simulink model "simcape_real_time_V2"  (R2022b)
settings: Solver=ode8  StartTime=0.0  StopTime=100  FixedStep=0.002  RelTol=1e-3
undefined symbols (not defined in the file): drone_leg, K_LQR, K_LQR_GOC, pitch_init, roll_init, v_pitch_init, v_roll_init, v_x_init, v_y_init, v_yaw_init, v_z_init, X, x_init, Y, y_init, yaw_init, Z, z_init
libraries: sm_lib x55, nesl_utility x12, simulink x7
(part 3 of 3)

== system simcape_real_time_V2/Subsystem4 ==
  Constant : Constant  Value=10
  Display : Display
  Subsystem : Subsystem
  Subsystem1 : Subsystem
  Subsystem3 : Subsystem
  Roll SP : Outport
  Pitch SP : Outport  Port=2
  wires:
  Subsystem/1(U1) -> Subsystem1/1(U1)
  Subsystem3/2(Pitch SP) -> Pitch SP/1
  Subsystem3/1(Roll SP) -> Roll SP/1
  [X_y] -> Subsystem1/3(y_SP)
  [X_x] -> Subsystem1/2(x_SP)
  Constant/1 -> Subsystem/1(z_SP)

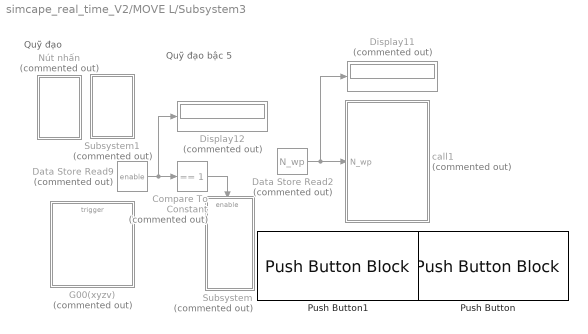
== system simcape_real_time_V2/MOVE L/Subsystem3 ==
  note: Quỹ đạo bậc 5
  note: Quỹ đạo
  Compare To Constant : simulink/Logic and Bit Operations/Compare To Constant  Commented=on  relop===  const=1  OutDataTypeStr=boolean
  Data Store Read2 : DataStoreRead  Commented=on  DataStoreName=N_wp  DataStoreElements=N_wp  IndexOptions=Index vector (dialog)  Indices=1  OutputSizes=1
  Data Store Read9 : DataStoreRead  Commented=on  DataStoreName=enable  IndexOptions=Index vector (dialog)  Indices=1  OutputSizes=1
  Display11 : Display  Commented=on
  Display12 : Display  Commented=on
  G00(xyzv) : Subsystem  Commented=on  TreatAsAtomicUnit=on
  Nút nhấn : Subsystem  Commented=on
  Push Button : PushButtonBlock  ButtonText=Start  IconColor=On  OffValue=0.000000
  Push Button1 : PushButtonBlock  ButtonText=Stop  IconColor=On  OffValue=0.000000
  Subsystem : Subsystem  Commented=on
  Subsystem1 : Subsystem  Commented=on
  call1 : MATLAB Function  Commented=on  TreatAsAtomicUnit=on
  wires:
  Data Store Read9/1 -> Display12/1, Compare To Constant/1
  Data Store Read2/1 -> Display11/1, call1/1(N_wp)
  Compare To Constant/1 -> Subsystem/Enable

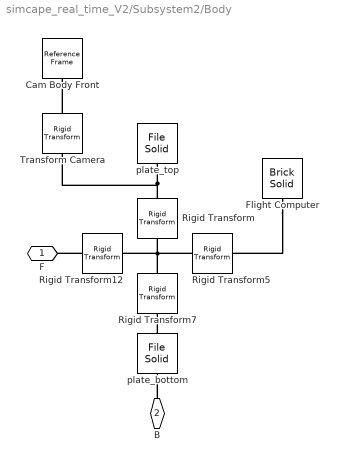
== system simcape_real_time_V2/Subsystem2/Body ==
  Cam Body Front : sm_lib/Frames and Transforms/Reference Frame
  Flight Computer : sm_lib/Body Elements/Brick Solid  GraphicAmbientColor=[0.15 0.15 0.15 1.0]  BasedOnType=Mass  BrickDimensions=3*[20 20 5]  BrickDimensionUnits=mm  CenterOfMass=[0 0 0]  CenterOfMassUnits=m  GraphicDiffuseColor=[0.5 0.5 0.5]  Density=1000  DensityUnits=kg/m^3  DoExposeReferenceFrame=on  GraphicEmissiveColor=[0.0 0.0 0.0 1.0]  ExportEntireGeometry=off  SerializedFrames=<Frames/>  MarkerShape=Sphere  MarkerSize=10  GraphicType=FromGeometry  InertiaType=CalculateFromGeometry  Mass=638  MassUnits=g  MomentsOfInertia=[1 1 1]  MomentsOfInertiaUnits=kg*m^2  GraphicOpacity=1.0  ProductsOfInertia=[0 0 0]  ProductsOfInertiaUnits=kg*m^2  GraphicShininess=75  GraphicSpecularColor=[0.5 0.5 0.5 1.0]  GraphicVisPropType=SimpleVisualProperties
  Rigid Transform : sm_lib/Frames and Transforms/Rigid Transform  TranslationMethod=None  TranslationStandardOffset=0  TranslationLengthUnit=m  TranslationStandardAxis=+Z  TranslationCartesianOffset=[0 0 0]  TranslationROffset=0  TranslationROffsetUnits=m  TranslationZOffset=0  TranslationZOffsetUnits=m  TranslationThetaOffset=0  TranslationThetaOffsetUnits=deg  RotationMethod=None  RotationAngleUnits=deg  RotationStandardAxis=+Z  RotationAngle=45  RotationArbitraryAxis=[0 0 1]  FollAlignAxisA=+X  BaseAlignAxisA=+Y  FollAlignAxisB=+Y  BaseAlignAxisB=+Z  RotationSequenceAxes=FollowerAxes  RotationSequence=XYX  RotationSequenceAngles=[0 0 0]  RotationSequenceAnglesUnits=deg  RotationMatrix=[1 0 0; 0 1 0; 0 0 1]  Quaternion=[1 0 0 0]
  Rigid Transform12 : sm_lib/Frames and Transforms/Rigid Transform  TranslationMethod=Cartesian  TranslationStandardOffset=0  TranslationLengthUnit=mm  TranslationStandardAxis=+Z  TranslationCartesianOffset=[0 0 -26]  TranslationROffset=0  TranslationROffsetUnits=m  TranslationZOffset=0  TranslationZOffsetUnits=m  TranslationThetaOffset=0  TranslationThetaOffsetUnits=deg  RotationMethod=None  RotationAngleUnits=deg  RotationStandardAxis=+Z  RotationAngle=45  RotationArbitraryAxis=[0 0 1]  FollAlignAxisA=+X  BaseAlignAxisA=+Y  FollAlignAxisB=+Y  BaseAlignAxisB=+Z  RotationSequenceAxes=FollowerAxes  RotationSequence=XYX  RotationSequenceAngles=[0 0 0]  RotationSequenceAnglesUnits=deg  RotationMatrix=[1 0 0; 0 1 0; 0 0 1]  Quaternion=[1 0 0 0]
  Rigid Transform5 : sm_lib/Frames and Transforms/Rigid Transform  TranslationMethod=Cartesian  TranslationStandardOffset=0  TranslationLengthUnit=mm  TranslationStandardAxis=+Z  TranslationCartesianOffset=[0 0 -26]  TranslationROffset=0  TranslationROffsetUnits=m  TranslationZOffset=0  TranslationZOffsetUnits=m  TranslationThetaOffset=0  TranslationThetaOffsetUnits=deg  RotationMethod=None  RotationAngleUnits=deg  RotationStandardAxis=+Z  RotationAngle=45  RotationArbitraryAxis=[0 0 1]  FollAlignAxisA=+X  BaseAlignAxisA=+Y  FollAlignAxisB=+Y  BaseAlignAxisB=+Z  RotationSequenceAxes=FollowerAxes  RotationSequence=XYX  RotationSequenceAngles=[0 0 0]  RotationSequenceAnglesUnits=deg  RotationMatrix=[1 0 0; 0 1 0; 0 0 1]  Quaternion=[1 0 0 0]
  Rigid Transform7 : sm_lib/Frames and Transforms/Rigid Transform  TranslationMethod=Cartesian  TranslationStandardOffset=0  TranslationLengthUnit=mm  TranslationStandardAxis=+Z  TranslationCartesianOffset=[0 0 -38]  TranslationROffset=0  TranslationROffsetUnits=m  TranslationZOffset=0  TranslationZOffsetUnits=m  TranslationThetaOffset=0  TranslationThetaOffsetUnits=deg  RotationMethod=None  RotationAngleUnits=deg  RotationStandardAxis=+Z  RotationAngle=45  RotationArbitraryAxis=[0 0 1]  FollAlignAxisA=+X  BaseAlignAxisA=+Y  FollAlignAxisB=+Y  BaseAlignAxisB=+Z  RotationSequenceAxes=FollowerAxes  RotationSequence=XYX  RotationSequenceAngles=[0 0 0]  RotationSequenceAnglesUnits=deg  RotationMatrix=[1 0 0; 0 1 0; 0 0 1]  Quaternion=[1 0 0 0]
  Transform Camera : sm_lib/Frames and Transforms/Rigid Transform  TranslationMethod=Cartesian  TranslationStandardOffset=0  TranslationLengthUnit=m  TranslationStandardAxis=+Z  TranslationCartesianOffset=[0.06 0 0]  TranslationROffset=0  TranslationROffsetUnits=m  TranslationZOffset=0  TranslationZOffsetUnits=m  TranslationThetaOffset=0  TranslationThetaOffsetUnits=deg  RotationMethod=None  RotationAngleUnits=deg  RotationStandardAxis=+Z  RotationAngle=0.0  RotationArbitraryAxis=[0 0 1]  FollAlignAxisA=+X  BaseAlignAxisA=+Y  FollAlignAxisB=+Y  BaseAlignAxisB=+Z  RotationSequenceAxes=FollowerAxes  RotationSequence=XYX  RotationSequenceAngles=[0 0 0]  RotationSequenceAnglesUnits=deg  RotationMatrix=[1 0 0; 0 1 0; 0 0 1]  Quaternion=[1 0 0 0]
  plate_bottom : sm_lib/Body Elements/File Solid  ExtGeomFileName=C:\Users\tridu\OneDrive\Máy tính\(1)\mohinh\quadcopter_simscape\Quadcopter-Simulation-master\Quadcopter-Simulation-master\CAD\Geometry\quadcopter_drone_plate_bottom.stp  UnitType=FromFile  ExtGeomFileUnits=m  StepReaderType=HEX  ExportConvexHullGeometry=off  InertiaType=Custom  Mass=0.0317292  MassUnits=kg  CenterOfMass=[9.57262e-08, 1.0716e-07, -1.47882e-10]  CenterOfMassUnits=m  MomentsOfInertia=[2.77785e-05, 2.75764e-05, 5.53432e-05]  MomentsOfInertiaUnits=kg*m^2  ProductsOfInertia=[-9.24719e-13, -9.71809e-13, 1.0181e-10]  ProductsOfInertiaUnits=kg*m^2  BasedOnType=Density  Density=1  DensityUnits=g/cm^3  DoExposeReferenceFrame=off  SerializedFrames=<Frames><Frame><Id>Frame1</Id><Value><Name>Bot</Name><Origin><Source>GeometricFeature</Source><FeatureName>planar surface 33</FeatureName></Origin><PrimaryAxis><DefinedDirection>+Z</DefinedDirection><Source>ReferenceFrame</Source><SourceDirection>+Z</SourceDirection><FeatureName></FeatureName></PrimaryAxis><SecondaryAxis><DefinedDirection>+X</DefinedDirection><Source>ReferenceFrame</Source><SourceDirection>+Y</SourceDirection><FeatureName></FeatureName></SecondaryAxis></Value></Frame><Frame><Id>Frame2</Id><Value><Name>Top</Name><Origin><Source>ReferenceFrame</Source><FeatureName></FeatureName></Origin><PrimaryAxis><DefinedDirection>+Z</DefinedDirection><Source>ReferenceFrame</Source><SourceDirection>+Z</SourceDirection><FeatureName></FeatureName></PrimaryAxis><SecondaryAxis><DefinedDirection>+X</DefinedDirection><Source>ReferenceFrame</Source><SourceDirection>+Y</SourceDirection><FeatureName></FeatureName></SecondaryAxis></Value></Frame></Frames>  GraphicType=FromGeometry  MarkerShape=Sphere  MarkerSize=10  GraphicVisPropType=SimpleVisualProperties  GraphicDiffuseColor=[0.0 0.0 0.0]  GraphicSpecularColor=[0.5 0.5 0.5 1.0]  GraphicAmbientColor=[0.15 0.15 0.15 1.0]  GraphicEmissiveColor=[0.0 0.0 0.0 1.0]  GraphicShininess=75  GraphicOpacity=1.0
  "plate_top " : sm_lib/Body Elements/File Solid  ExtGeomFileName=C:\Users\tridu\OneDrive\Máy tính\(1)\mohinh\quadcopter_simscape\Quadcopter-Simulation-master\Quadcopter-Simulation-master\CAD\Geometry\quadcopter_drone_plate_top.stp  UnitType=FromFile  ExtGeomFileUnits=m  StepReaderType=HEX  ExportConvexHullGeometry=off  InertiaType=Custom  Mass=0.0317292  MassUnits=kg  CenterOfMass=[9.57262e-08, 1.0716e-07, -1.47882e-10]  CenterOfMassUnits=m  MomentsOfInertia=[2.77785e-05, 2.75764e-05, 5.53432e-05]  MomentsOfInertiaUnits=kg*m^2  ProductsOfInertia=[-9.24719e-13, -9.71809e-13, 1.0181e-10]  ProductsOfInertiaUnits=kg*m^2  BasedOnType=Density  Density=1  DensityUnits=g/cm^3  DoExposeReferenceFrame=on  SerializedFrames=<Frames/>  GraphicType=FromGeometry  MarkerShape=Sphere  MarkerSize=10  GraphicVisPropType=SimpleVisualProperties  GraphicDiffuseColor=[0.0 0.0 0.0]  GraphicSpecularColor=[0.5 0.5 0.5 1.0]  GraphicAmbientColor=[0.15 0.15 0.15 1.0]  GraphicEmissiveColor=[0.0 0.0 0.0 1.0]  GraphicShininess=75  GraphicOpacity=1.0
  F : PMIOPort  Side=Right
  B : PMIOPort  Port=2  Side=Left
  connections:
  Flight Computer/RConn1 -- Rigid Transform5/RConn1
  Rigid Transform7/LConn1 -- Rigid Transform5/LConn1 -- Rigid Transform12/LConn1 -- Rigid Transform/LConn1
  plate_bottom/RConn1 -- Rigid Transform7/RConn1
  Rigid Transform12/RConn1 -- F/RConn1
  Rigid Transform/RConn1 -- Transform Camera/LConn1 -- "plate_top "/RConn1
  Transform Camera/RConn1 -- Cam Body Front/RConn1
  B/RConn1 -- plate_bottom/LConn1

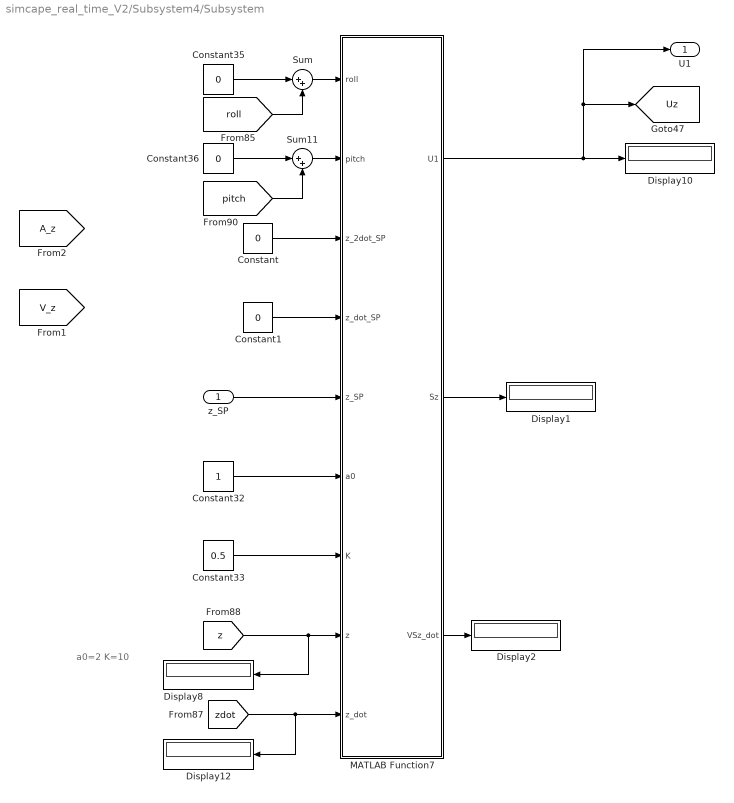
== system simcape_real_time_V2/Subsystem4/Subsystem ==
  note: a0=2
      | K=10
  z_SP : Inport
  Constant{,1,35..36} (4 alike) : Constant  Value=0
  Constant32 : Constant
  Constant33 : Constant  Value=0.5
  Display{1..2,8,10,12} (5 alike) : Display
  MATLAB Function7 : MATLAB Function  TreatAsAtomicUnit=on
  Sum : Sum  Inputs=|++
  Sum11 : Sum  Inputs=|++
  U1 : Outport
  tag scope: Uz=global
  wires:
  [z] -> Display8/1, MATLAB Function7/8(z)
  Constant35/1 -> Sum/1
  Constant32/1 -> MATLAB Function7/6(a0)
  [zdot] -> Display12/1, MATLAB Function7/9(z_dot)
  Sum11/1 -> MATLAB Function7/2(pitch)
  [roll] -> Sum/2
  Constant33/1 -> MATLAB Function7/7(K)
  [pitch] -> Sum11/2
  Sum/1 -> MATLAB Function7/1(roll)
  MATLAB Function7/1(U1) -> U1/1, [Uz], Display10/1
  Constant36/1 -> Sum11/1
  MATLAB Function7/2(Sz) -> Display1/1
  MATLAB Function7/3(VSz_dot) -> Display2/1
  z_SP/1 -> MATLAB Function7/5(z_SP)
  Constant/1 -> MATLAB Function7/3(z_2dot_SP)
  Constant1/1 -> MATLAB Function7/4(z_dot_SP)

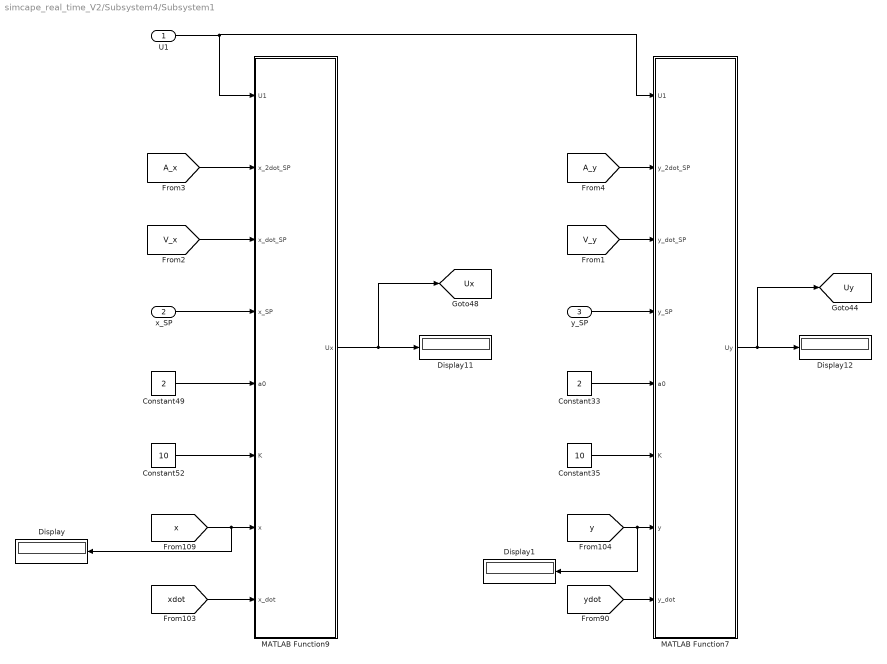
== system simcape_real_time_V2/Subsystem4/Subsystem1 ==
  U1 : Inport
  x_SP : Inport  Port=2
  y_SP : Inport  Port=3
  Constant33 : Constant  Value=2
  Constant35 : Constant  Value=10
  Constant49 : Constant  Value=2
  Constant52 : Constant  Value=10
  Display{,1,11..12} (4 alike) : Display
  MATLAB Function7 : MATLAB Function  TreatAsAtomicUnit=on
  MATLAB Function9 : MATLAB Function  TreatAsAtomicUnit=on
  tag scope: Ux=global, Uy=global
  wires:
  Constant49/1 -> MATLAB Function9/5(a0)
  [x] -> Display/1, MATLAB Function9/7(x)
  Constant52/1 -> MATLAB Function9/6(K)
  [xdot] -> MATLAB Function9/8(x_dot)
  x_SP/1 -> MATLAB Function9/4(x_SP)
  MATLAB Function9/1(Ux) -> [Ux], Display11/1
  y_SP/1 -> MATLAB Function7/4(y_SP)
  U1/1 -> MATLAB Function7/1(U1), MATLAB Function9/1(U1)
  [ydot] -> MATLAB Function7/8(y_dot)
  Constant33/1 -> MATLAB Function7/5(a0)
  Constant35/1 -> MATLAB Function7/6(K)
  MATLAB Function7/1(Uy) -> [Uy], Display12/1
  [V_x] -> MATLAB Function9/3(x_dot_SP)
  [A_x] -> MATLAB Function9/2(x_2dot_SP)
  [V_y] -> MATLAB Function7/3(y_dot_SP)
  [A_y] -> MATLAB Function7/2(y_2dot_SP)
  [y] -> Display1/1, MATLAB Function7/7(y)

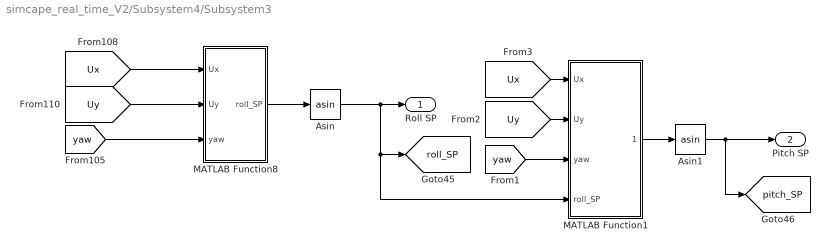
== system simcape_real_time_V2/Subsystem4/Subsystem3 ==
  Asin : Trigonometry  Operator=asin
  Asin1 : Trigonometry  Operator=asin
  MATLAB Function1 : MATLAB Function  TreatAsAtomicUnit=on
  MATLAB Function8 : MATLAB Function  TreatAsAtomicUnit=on
  Roll SP : Outport
  Pitch SP : Outport  Port=2
  tag scope: pitch_SP=global, roll_SP=global
  wires:
  [Ux] -> MATLAB Function8/1(Ux)
  [Uy] -> MATLAB Function8/2(Uy)
  MATLAB Function8/1(roll_SP) -> Asin/1
  Asin/1 -> Roll SP/1, MATLAB Function1/4(roll_SP), [roll_SP]
  [yaw] -> MATLAB Function8/3(yaw)
  [yaw] -> MATLAB Function1/3(yaw)
  [Uy] -> MATLAB Function1/2(Uy)
  [Ux] -> MATLAB Function1/1(Ux)
  Asin1/1 -> [pitch_SP], Pitch SP/1
  MATLAB Function1/1(pitch_SP) -> Asin1/1

== system simcape_real_time_V2/MOVE L/Subsystem3/G00(xyzv) ==
  G00 : TriggerPort  TriggerType=function-call  IsSimulinkFunction=on  FunctionName=G00  FunctionVisibility=scoped  VariantControl=(inherit)
  Data Store Write2 : DataStoreWrite  DataStoreName=xyzv  IndexOptions=Index vector (dialog)  Indices=1  OutputSizes=1
  Display : Display
  Display1 : Display
  MATLAB Function1 : MATLAB Function  TreatAsAtomicUnit=on
  xyzv : ArgIn  DisableCoverage=on  PortDimensions=4  ArgumentName=xyzv
  wires:
  MATLAB Function1/1(xyzv_out) -> Display/1, Data Store Write2/1
  xyzv/1 -> Display1/1, MATLAB Function1/1(xyzv_in)

== system simcape_real_time_V2/MOVE L/Subsystem3/Nút nhấn ==
  Compare To Constant10 : simulink/Logic and Bit Operations/Compare To Constant  relop===  const=1  OutDataTypeStr=boolean
  Constant5 : Constant  Value=0
  Data Store Read1 : DataStoreRead  DataStoreName=start  DataStoreElements=start  IndexOptions=Index vector (dialog)  Indices=1  OutputSizes=1
  Data Store Write : DataStoreWrite  DataStoreName=start  IndexOptions=Index vector (dialog)  Indices=1  OutputSizes=1
  START : Subsystem  TreatAsAtomicUnit=on
  wires:
  Compare To Constant10/1 -> START/Trigger
  Data Store Read1/1 -> Compare To Constant10/1
  Constant5/1 -> Data Store Write/1

== system simcape_real_time_V2/MOVE L/Subsystem3/Subsystem ==
  Enable : EnablePort
  Quỹ đạo bậc 5 : Subsystem

== system simcape_real_time_V2/MOVE L/Subsystem3/Subsystem1 ==
  Compare To Constant : simulink/Logic and Bit Operations/Compare To Constant  relop===  const=1  OutDataTypeStr=boolean
  Compare To Constant1 : simulink/Logic and Bit Operations/Compare To Constant  relop===  const=0  OutDataTypeStr=boolean
  Data Store Read : DataStoreRead  DataStoreName=stop  IndexOptions=Index vector (dialog)  Indices=1  OutputSizes=1
  Data Store Write : DataStoreWrite  DataStoreName=stop  IndexOptions=Index vector (dialog)  Indices=1  OutputSizes=1
  Stop : Constant  Value=0
  Triggered Subsystem : Subsystem  TreatAsAtomicUnit=on
  Triggered Subsystem1 : Subsystem  TreatAsAtomicUnit=on
  wires:
  Stop/1 -> Data Store Write/1
  Data Store Read/1 -> Compare To Constant/1
  Compare To Constant/1 -> Triggered Subsystem/Trigger
  [z] -> Compare To Constant1/1
  Compare To Constant1/1 -> Triggered Subsystem1/Trigger

== system simcape_real_time_V2/MOVE L/Subsystem3/Nút nhấn/START ==
  Trigger : TriggerPort  VariantControl=Variant  InitialTriggerSignalState=zero  PortDimensions=1
  Compare To Constant : simulink/Logic and Bit Operations/Compare To Constant  relop===  const=0  OutDataTypeStr=boolean
  Constant : Constant
  Constant1 : Constant
  Constant2 : Constant  Value=-1
  Data Store Read : DataStoreRead  DataStoreName=N_wp  IndexOptions=Index vector (dialog)  Indices=1  OutputSizes=1
  Data Store Write : DataStoreWrite  DataStoreName=motor_13  IndexOptions=Index vector (dialog)  Indices=1  OutputSizes=1
  Data Store Write1 : DataStoreWrite  DataStoreName=enable  IndexOptions=Index vector (dialog)  Indices=1  OutputSizes=1
  Data Store Write2 : DataStoreWrite  DataStoreName=motor_24  IndexOptions=Index vector (dialog)  Indices=1  OutputSizes=1
  Subsystem : Subsystem
  wires:
  Compare To Constant/1 -> Subsystem/Enable
  Data Store Read/1 -> Compare To Constant/1
  Constant/1 -> Data Store Write1/1
  Constant1/1 -> Data Store Write/1
  Constant2/1 -> Data Store Write2/1

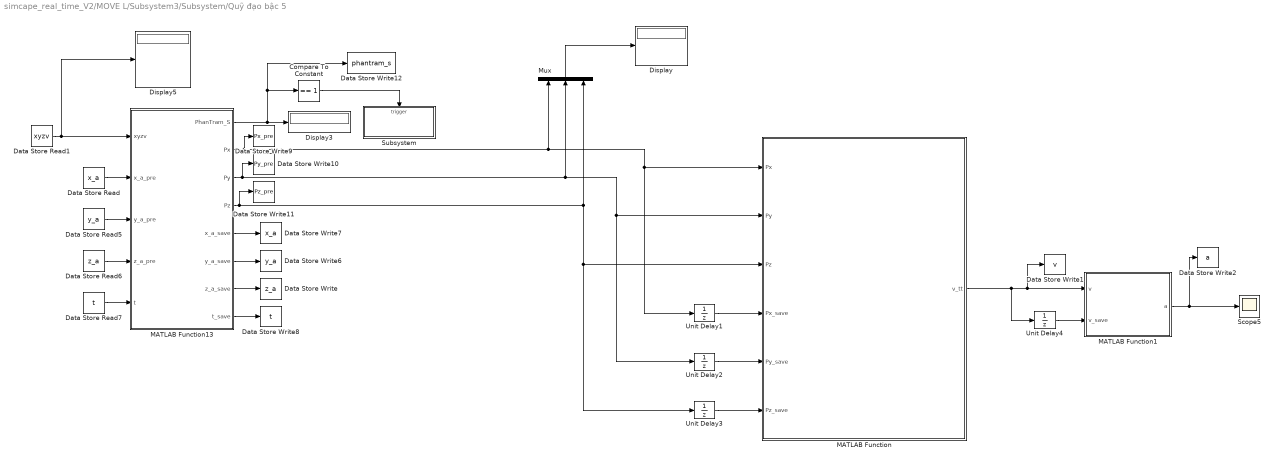
== system simcape_real_time_V2/MOVE L/Subsystem3/Subsystem/Quỹ đạo bậc 5 ==
  Compare To Constant : simulink/Logic and Bit Operations/Compare To Constant  relop===  const=1  OutDataTypeStr=boolean
  Data Store Read : DataStoreRead  DataStoreName=x_a  IndexOptions=Index vector (dialog)  Indices=1  OutputSizes=1
  Data Store Read1 : DataStoreRead  DataStoreName=xyzv  IndexOptions=Index vector (dialog)  Indices=1  OutputSizes=1
  Data Store Read5 : DataStoreRead  DataStoreName=y_a  IndexOptions=Index vector (dialog)  Indices=1  OutputSizes=1
  Data Store Read6 : DataStoreRead  DataStoreName=z_a  IndexOptions=Index vector (dialog)  Indices=1  OutputSizes=1
  Data Store Read7 : DataStoreRead  DataStoreName=t  IndexOptions=Index vector (dialog)  Indices=1  OutputSizes=1
  Data Store Write : DataStoreWrite  DataStoreName=z_a  IndexOptions=Index vector (dialog)  Indices=1  OutputSizes=1
  Data Store Write1 : DataStoreWrite  DataStoreName=v  IndexOptions=Index vector (dialog)  Indices=1  OutputSizes=1
  Data Store Write10 : DataStoreWrite  DataStoreName=Py_pre  IndexOptions=Index vector (dialog)  Indices=1  OutputSizes=1
  Data Store Write11 : DataStoreWrite  DataStoreName=Pz_pre  IndexOptions=Index vector (dialog)  Indices=1  OutputSizes=1
  Data Store Write12 : DataStoreWrite  DataStoreName=phantram_s  DataStoreElements=phantram_s  IndexOptions=Index vector (dialog)  Indices=1  OutputSizes=1
  Data Store Write2 : DataStoreWrite  DataStoreName=a  IndexOptions=Index vector (dialog)  Indices=1  OutputSizes=1
  Data Store Write6 : DataStoreWrite  DataStoreName=y_a  IndexOptions=Index vector (dialog)  Indices=1  OutputSizes=1
  Data Store Write7 : DataStoreWrite  DataStoreName=x_a  IndexOptions=Index vector (dialog)  Indices=1  OutputSizes=1
  Data Store Write8 : DataStoreWrite  DataStoreName=t  IndexOptions=Index vector (dialog)  Indices=1  OutputSizes=1
  Data Store Write9 : DataStoreWrite  DataStoreName=Px_pre  IndexOptions=Index vector (dialog)  Indices=1  OutputSizes=1
  Display : Display
  Display3 : Display
  Display5 : Display
  MATLAB Function : MATLAB Function  TreatAsAtomicUnit=on
  MATLAB Function1 : MATLAB Function  TreatAsAtomicUnit=on
  MATLAB Function13 : MATLAB Function  TreatAsAtomicUnit=on
  Mux : Mux  Inputs=3
  Scope5 : Scope
  Subsystem : Subsystem
  Unit Delay{1..4} (4 alike) : UnitDelay  SampleTime=-1  HasFrameUpgradeWarning=on
  wires:
  MATLAB Function13/8(t_save) -> Data Store Write8/1
  Compare To Constant/1 -> Subsystem/Trigger
  MATLAB Function13/1(PhanTram_S) -> Data Store Write12/1, Compare To Constant/1, Display3/1
  Data Store Read/1 -> MATLAB Function13/2(x_a_pre)
  Data Store Read6/1 -> MATLAB Function13/4(z_a_pre)
  MATLAB Function13/7(z_a_save) -> Data Store Write/1
  Data Store Read1/1 -> Display5/1, MATLAB Function13/1(xyzv)
  MATLAB Function13/5(x_a_save) -> Data Store Write7/1
  MATLAB Function13/6(y_a_save) -> Data Store Write6/1
  Data Store Read7/1 -> MATLAB Function13/5(t)
  Data Store Read5/1 -> MATLAB Function13/3(y_a_pre)
  Unit Delay4/1 -> MATLAB Function1/2(v_save)
  MATLAB Function13/3(Py) -> MATLAB Function/2(Py), Unit Delay2/1, Mux/2, Data Store Write10/1
  Unit Delay2/1 -> MATLAB Function/5(Py_save)
  MATLAB Function13/4(Pz) -> Mux/3, MATLAB Function/3(Pz), Unit Delay3/1, Data Store Write11/1
  MATLAB Function/1(v_tt) -> Unit Delay4/1, Data Store Write1/1, MATLAB Function1/1(v)
  MATLAB Function13/2(Px) -> Unit Delay1/1, MATLAB Function/1(Px), Mux/1, Data Store Write9/1
  Unit Delay1/1 -> MATLAB Function/4(Px_save)
  MATLAB Function1/1(a) -> Data Store Write2/1, Scope5/1
  Unit Delay3/1 -> MATLAB Function/6(Pz_save)
  Mux/1 -> Display/1

== system simcape_real_time_V2/MOVE L/Subsystem3/Subsystem1/Triggered Subsystem ==
  Trigger : TriggerPort  VariantControl=(inherit)
  Constant : Constant  Value=0
  Constant1 : Constant  Value=0
  Constant2 : Constant  Value=0
  Data Store Write : DataStoreWrite  DataStoreName=enable  IndexOptions=Index vector (dialog)  Indices=1  OutputSizes=1
  Data Store Write1 : DataStoreWrite  DataStoreName=N_wp  IndexOptions=Index vector (dialog)  Indices=1  OutputSizes=1
  Data Store Write2 : DataStoreWrite  DataStoreName=Px_pre  IndexOptions=Index vector (dialog)  Indices=1  OutputSizes=1
  Data Store Write3 : DataStoreWrite  DataStoreName=Py_pre  IndexOptions=Index vector (dialog)  Indices=1  OutputSizes=1
  Data Store Write4 : DataStoreWrite  DataStoreName=Pz_pre  IndexOptions=Index vector (dialog)  Indices=1  OutputSizes=1
  wires:
  Constant/1 -> Data Store Write/1
  Constant1/1 -> Data Store Write1/1
  Constant2/1 -> Data Store Write4/1, Data Store Write3/1, Data Store Write2/1

== system simcape_real_time_V2/MOVE L/Subsystem3/Subsystem1/Triggered Subsystem1 ==
  Trigger : TriggerPort  VariantControl=(inherit)
  Constant : Constant  Value=0
  Data Store Write : DataStoreWrite  DataStoreName=motor_13  IndexOptions=Index vector (dialog)  Indices=1  OutputSizes=1
  Data Store Write1 : DataStoreWrite  DataStoreName=motor_24  IndexOptions=Index vector (dialog)  Indices=1  OutputSizes=1
  wires:
  Constant/1 -> Data Store Write1/1, Data Store Write/1

== system simcape_real_time_V2/MOVE L/Subsystem3/Nút nhấn/START/Subsystem ==
  Enable : EnablePort
  Constant1 : Constant
  Data Store Write1 : DataStoreWrite  DataStoreName=N_wp  DataStoreElements=N_wp  IndexOptions=Index vector (dialog)  Indices=1  OutputSizes=1
  wires:
  Constant1/1 -> Data Store Write1/1

== system simcape_real_time_V2/MOVE L/Subsystem3/Subsystem/Quỹ đạo bậc 5/Subsystem ==
  Trigger : TriggerPort  VariantControl=Variant  PortDimensions=1
  Add : Sum
  Constant : Constant  OutDataTypeStr=double
  Data Store Read : DataStoreRead  DataStoreName=N_wp  DataStoreElements=N_wp  IndexOptions=Index vector (dialog)  Indices=1  OutputSizes=1
  Data Store Write : DataStoreWrite  DataStoreName=N_wp  DataStoreElements=N_wp  IndexOptions=Index vector (dialog)  Indices=1  OutputSizes=1
  Display : Display
  wires:
  Constant/1 -> Add/2
  Data Store Read/1 -> Add/1
  Add/1 -> Display/1, Data Store Write/1

== matlab function simcape_real_time_V2/MATLAB Function2 ==
  data: T1 input; D1 output; T2 input; T3 input; T4 input; D2 output; D3 output; D4 output
function [D1,D2,D3,D4]= fcn(T1,T2,T3,T4)
D1=(T1/11.5)*1000+1000;
D2=(T2/11.5)*1000+1000;
D3=(T3/11.5)*1000+1000;
D4=(T4/11.5)*1000+1000;

end

== matlab function simcape_real_time_V2/Subsystem4/Subsystem3/MATLAB Function1 ==
  data: Ux input; pitch_SP output; Uy input; yaw input; roll_SP input
function pitch_SP = fcn(Ux,Uy,yaw,roll_SP)

pitch_SP=(cos(yaw)*Ux+sin(yaw)*Uy)/cos(roll_SP);

end

== matlab function simcape_real_time_V2/Quỹ đạo trục z/MATLAB Function10 ==
  data: q0 input; X output; qf input; v_qd input; V output; A output
function [X,V,A]= fcn(q0,qf,v_qd)
persistent t  a0 a1 a2 a3 a4 a5 

ts=0.002; %% thời gian lấy mẫu 

tf   = qf/v_qd; %% thời gian hoàn thành quãng đường

%% Quy hoạch quỹ đạo đa thức bậc 5

v0=0; % vận tốc nam đầu
ao=0; % gia tốc ban đầu

vf=0;   % vận tốc điểm cuối
af=0;   % gia tốc điểm cuối

a0 = q0;
a1 = v0;
a2 = ao/2;
a3 = -(20*q0 - 20*qf + 12*v0*tf + 8*vf*tf + 3*ao*tf^2 - af*tf^2)/(2*tf^3);
a4 = (30*q0 - 30*qf + 16*v0*tf + 14*vf*tf + 3*ao*tf^2 - 2*af*tf^2)/(2*tf^4);
a5 = -(12*q0 - 12*qf + 6*v0*tf + 6*vf*tf + ao*tf^2 - af*tf^2)/(2*tf^5);
          

if isempty(t)    
    t = 0;
end
%% thời gian ban đầu
    t = t + ts;
%     t_out = t;
 %% Check điều kiện dừng
if(t>tf)
    t=tf;
end

%% công thức tổng quát quỹ đạo bậc 5 vị trí theo thời gian t
X= a0 + a1*t + a2*t^2 + a3*t^3 + a4*t^4 + a5*t^5;
%% công thức tổng quát quỹ đạo bậc 5 vị trí theo thời gian t
V= a1 + 2*a2*t + 3*a3*t^2 + 4*a4*t^3 + 5*a5*t^4;
%% công thức tổng quát quỹ đạo bậc 5 vị trí theo thời gian t
A=  2*a2 + 6*a3*t + 12*a4*t^2 + 20*a5*t^3;
if(qf==0)
  X=0;
  V=0;
  A=0;
 end
end

== matlab function simcape_real_time_V2/Quỹ đạo trục x/MATLAB Function10 ==
  data: q0 input; X output; qf input; v_qd input; V output; A output
function [X,V,A]= fcn(q0,qf,v_qd)
persistent t  a0 a1 a2 a3 a4 a5 

ts=0.002; %% thời gian lấy mẫu 

tf   = qf/v_qd; %% thời gian hoàn thành quãng đường

%% Quy hoạch quỹ đạo đa thức bậc 5

v0=0; % vận tốc nam đầu
ao=0; % gia tốc ban đầu

vf=0;   % vận tốc điểm cuối
af=0;   % gia tốc điểm cuối

a0 = q0;
a1 = v0;
a2 = ao/2;
a3 = -(20*q0 - 20*qf + 12*v0*tf + 8*vf*tf + 3*ao*tf^2 - af*tf^2)/(2*tf^3);
a4 = (30*q0 - 30*qf + 16*v0*tf + 14*vf*tf + 3*ao*tf^2 - 2*af*tf^2)/(2*tf^4);
a5 = -(12*q0 - 12*qf + 6*v0*tf + 6*vf*tf + ao*tf^2 - af*tf^2)/(2*tf^5);
          

if isempty(t)    
    t = 0;
end
%% thời gian ban đầu
    t = t + ts;
%     t_out = t;
 %% Check điều kiện dừng
if(t>tf)
    t=tf;
end

%% công thức tổng quát quỹ đạo bậc 5 vị trí theo thời gian t
X= a0 + a1*t + a2*t^2 + a3*t^3 + a4*t^4 + a5*t^5;
%% công thức tổng quát quỹ đạo bậc 5 vị trí theo thời gian t
V= a1 + 2*a2*t + 3*a3*t^2 + 4*a4*t^3 + 5*a5*t^4;
%% công thức tổng quát quỹ đạo bậc 5 vị trí theo thời gian t
A=  2*a2 + 6*a3*t + 12*a4*t^2 + 20*a5*t^3;
if(qf==0)
  X=0;
  V=0;
  A=0;
 end
end

== matlab function simcape_real_time_V2/Quỹ đạo trục y/MATLAB Function10 ==
  data: q0 input; X output; qf input; v_qd input; V output; A output
function [X,V,A]= fcn(q0,qf,v_qd)
persistent t  a0 a1 a2 a3 a4 a5 

ts=0.002; %% thời gian lấy mẫu 

tf   = qf/v_qd; %% thời gian hoàn thành quãng đường


%% Quy hoạch quỹ đạo đa thức bậc 5

v0=0; % vận tốc nam đầu
ao=0; % gia tốc ban đầu

vf=0;   % vận tốc điểm cuối
af=0;   % gia tốc điểm cuối

a0 = q0;
a1 = v0;
a2 = ao/2;
a3 = -(20*q0 - 20*qf + 12*v0*tf + 8*vf*tf + 3*ao*tf^2 - af*tf^2)/(2*tf^3);
a4 = (30*q0 - 30*qf + 16*v0*tf + 14*vf*tf + 3*ao*tf^2 - 2*af*tf^2)/(2*tf^4);
a5 = -(12*q0 - 12*qf + 6*v0*tf + 6*vf*tf + ao*tf^2 - af*tf^2)/(2*tf^5);
          

if isempty(t)    
    t = 0;
end
%% thời gian ban đầu
    t = t + ts;
%     t_out = t;
 %% Check điều kiện dừng
if(t>tf)
    t=tf;
end

%% công thức tổng quát quỹ đạo bậc 5 vị trí theo thời gian t
X= a0 + a1*t + a2*t^2 + a3*t^3 + a4*t^4 + a5*t^5;
%% công thức tổng quát quỹ đạo bậc 5 vị trí theo thời gian t
V= a1 + 2*a2*t + 3*a3*t^2 + 4*a4*t^3 + 5*a5*t^4;
%% công thức tổng quát quỹ đạo bậc 5 vị trí theo thời gian t
A=  2*a2 + 6*a3*t + 12*a4*t^2 + 20*a5*t^3;

if(qf==0)
  X=0;
  V=0;
  A=0;
 end
end

== matlab function simcape_real_time_V2/MOVE L/Subsystem3/G00(xyzv)/MATLAB Function1 ==
  data: xyzv_in input; xyzv_out output
function xyzv_out = fcn(xyzv_in)
        
        x_out = xyzv_in(1);
        y_out = xyzv_in(2);
        z_out = xyzv_in(3);
        v_out = xyzv_in(4);
        
        xyzv_out  = [x_out ; y_out ; z_out ; v_out ];
end

== matlab function simcape_real_time_V2/Subsystem4/Subsystem/MATLAB Function7 ==
  settings: updateMethod=DISCRETE
  data: roll input; pitch input; z_2dot_SP input; z_dot_SP input; z_SP input; a0 input; K input; z input; z_dot input; U1 output; Sz output; VSz_dot output
function [U1,Sz,VSz_dot]= fcn(roll,pitch,z_2dot_SP,z_dot_SP,z_SP,a0,K,z,z_dot)  
    %% khai báo biến hệ thống
    g=9.81;
    m=1.7;
    %% phương trình trạng thái
    % z_2dot=((U1*cos(pitch)*cos(roll))/m) - g;
    %% Chọn phương trình mặt trượt có dạng
    Sz=(z_dot_SP-z_dot)+a0*(z_SP-z);
    %% Chọn tiêu chí tốc độ hội tụ, trong đó K là hệ số dương Nếu K càng lớn thì độ hội tụ về 0 càng giảm
    VSz_dot=-K*sign(Sz);
    %% Thiết kế tín hiệu điều khiển Ux Uy
    U1=(m/(cos(roll)*cos(pitch)))*(z_2dot_SP+K*sign(Sz)*abs(Sz)+g+a0*(z_dot_SP-z_dot));
end

== matlab function simcape_real_time_V2/Subsystem4/Subsystem1/MATLAB Function7 ==
  data: U1 input; y_2dot_SP input; y_dot_SP input; y_SP input; a0 input; Uy output; K input; y input; y_dot input
function Uy = fcn(U1,y_2dot_SP,y_dot_SP,y_SP,a0,K,y,y_dot) 

%% khai báo biến hệ thống
m=1.7;

%% phương trình trạng thái

% y_2dot=-(U1*cos(yaw)*sin(roll) - cos(roll)*sin(pitch)*sin(yaw))/m;

%% Chọn phương trình mặt trượt có dạng

Sy=(y_dot_SP-y_dot)+a0*(y_SP-y);

%% Chọn tiêu chí tốc độ hội tụ, trong đó K là hệ số dương Nếu K càng lớn thì độ hội tụ về 0 càng giảm

VSy=-K*sign(Sy);

%% Thiết kế tín hiệu điều khiển Ux Uy

Uy=(m/U1)*(y_2dot_SP+a0*(y_dot_SP-y_dot)+K*sign(Sy)*abs(Sy));

end

== matlab function simcape_real_time_V2/Subsystem4/Subsystem1/MATLAB Function9 ==
  data: U1 input; x_2dot_SP input; x_dot_SP input; x_SP input; a0 input; K input; Ux output; x input; x_dot input
function Ux = fcn(U1,x_2dot_SP,x_dot_SP,x_SP,a0,K,x,x_dot) 

%% khai báo biến hệ thống

m=1.7;

%% phương trình trạng thái

% x_2dot=(U1*sin(roll)*sin(yaw) + cos(roll)*cos(yaw)*sin(pitch))/m;

%% Chọn phương trình mặt trượt có dạng

Sx=(x_dot_SP-x_dot)+a0*(x_SP-x);

%% Chọn tiêu chí tốc độ hội tụ, trong đó K là hệ số dương Nếu K càng lớn thì độ hội tụ về 0 càng giảm

VSx=-K*sign(Sx);

%% Thiết kế tín hiệu điều khiển Ux Uy

Ux=(m/U1)*(x_2dot_SP+a0*(x_dot_SP-x_dot)+K*sign(Sx)*abs(Sx));

end

== matlab function simcape_real_time_V2/Subsystem4/Subsystem3/MATLAB Function8 ==
  data: Ux input; roll_SP output; Uy input; yaw input
function roll_SP = fcn(Ux,Uy,yaw)

roll_SP=(sin(yaw)*Ux)-(cos(yaw)*Uy);

end

== matlab function simcape_real_time_V2/MOVE L/Subsystem3/Subsystem/Quỹ đạo bậc 5/MATLAB Function13 ==
  data: xyzv input; PhanTram_S output; Px output; Py output; Pz output; x_a_save output; y_a_save output; z_a_save output; t_save output; x_a_pre input; y_a_pre input; z_a_pre input; t input
function [PhanTram_S,Px,Py,Pz,x_a_save,y_a_save,z_a_save,t_save]= fcn(xyzv,x_a_pre,y_a_pre,z_a_pre,t)
    x_b=xyzv(1);
    y_b=xyzv(2);
    z_b=xyzv(3);
    v_tb=xyzv(4);
    AB = sqrt((x_b-x_a_pre)^2+(y_b-y_a_pre)^2+(z_b-z_a_pre)^2);
    if(v_tb>0)
        tf = AB/v_tb;
    else
        tf=0;
    end
    ts = 0.002; 
    %% Nội suy Phần tram quãng đường liên tục theo thời gian theo phương pháp quy hoạch quỹ đạo bậc 3
    a_0 = 0;
    a_1 = 0;
    a_2 = 0;
    a_3 = ((20*AB)/(2*tf*tf*tf));
    a_4 = ((-30*AB)/(2*tf*tf*tf*tf));
    a_5 = ((12*AB)/(2*tf*tf*tf*tf*tf));
    if(t<tf)
        t_save=t+ts;
        temp=0;
    elseif(t>=tf)
        t_save=0;
        temp=1;
     else
        t_save=t;
        temp=0;
     end
    if(AB<=0)&&(temp==1)
        PhanTram_S = 1;
    else
        PhanTram_S=((a_0+ (a_1*t) + (a_2*t*t) + (a_3*t*t*t) + (a_4*t*t*t*t) + (a_5*t*t*t*t*t))/AB);
    end
     %%%

    %% Nội suy tọa độ theo công thức hình học.
    if(temp==1)
        Px=x_b;
        Py=y_b;
        Pz=z_b;
        x_a_save=x_b;
        y_a_save=y_b;
        z_a_save=z_b; 
    else
        x_a_save=x_a_pre;
        y_a_save=y_a_pre;
        z_a_save=z_a_pre;
        Px = x_a_pre + (x_b-x_a_pre)*PhanTram_S;
        Py = y_a_pre + (y_b-y_a_pre)*PhanTram_S;
        Pz = z_a_pre + (z_b-z_a_pre)*PhanTram_S;
    end
    % vx=(Px-Px_save)/ts;
    % vy=(Py-Py_save)/ts;
    % vz=(Pz-Pz_save)/ts;
    % v_tt=sqrt(vx*vx+vy*vy+vz*vz);
    % a_tt=(v_tt - v_tt_save)/ts;
    % Px_save=Px;
    % Py_save=Py;
    % Pz_save=Pz;
    % v_tt_save=v_tt;
     
end

== matlab function simcape_real_time_V2/MOVE L/Subsystem3/call1 ==
  data: N_wp input
function fcn(N_wp)
    switch(N_wp)  
        case 1
        G00([0;0;100;50]);
        case 2
        G00([-280;0;100;10]);
        case 3
        G00([-280;-280;100;10]);
        case 4
        G00([0;-280;100;10]);
        case 5
        G00([0;0;100;10]);
        case 6
        G00([0;0;0;50]);        
    end
end

== matlab function simcape_real_time_V2/MOVE L/Subsystem3/Subsystem/Quỹ đạo bậc 5/MATLAB Function ==
  data: Px input; v_tt output; Py input; Pz input; Px_save input; Py_save input; Pz_save input
function v_tt = fcn(Px,Py,Pz,Px_save,Py_save,Pz_save)
  ts=0.002;
  vx=(Px-Px_save)/ts;
  vy=(Py-Py_save)/ts;
  vz=(Pz-Pz_save)/ts;
  v_tt=sqrt((vx*vx)+(vy*vy)+(vz*vz));
end

== matlab function simcape_real_time_V2/MOVE L/Subsystem3/Subsystem/Quỹ đạo bậc 5/MATLAB Function1 ==
  data: v input; a output; v_save input
function a = fcn(v,v_save)
    ts=0.002;
    a=(v-v_save)/ts;
end

== matlab function simcape_real_time_V2/MATLAB Function1 ==
  data: D1 input; T1 output; D2 input; D3 input; D4 input; T2 output; T3 output; T4 output
function [T1,T2,T3,T4]= fcn(D1,D2,D3,D4)
T1=(D1-1000)/1000*11.5;
T2=(D2-1000)/1000*11.5;
T3=(D3-1000)/1000*11.5;
T4=(D4-1000)/1000*11.5;

end

== matlab function simcape_real_time_V2/MATLAB Function ==
  data: T1 input; x2dot output; T2 input; T3 input; T4 input; roll input; pitch input; yaw input; roll_dot input; pitch_dot input; yaw_dot input; y2dot output; z2dot output; roll2dot output; pitch2dot output; yaw2dot output; HS_MSKK input; x_dot input; y_dot input; z_dot input
function [x2dot,y2dot,z2dot,roll2dot,pitch2dot,yaw2dot]= fcn(T1,T2,T3,T4,roll,pitch,yaw,roll_dot,pitch_dot,yaw_dot,HS_MSKK,x_dot,y_dot,z_dot)
    m = 1.7; %kg
    l = 0.25; %m
    % % b = 4.74E-5;
    % % d = 2.35E-7;
    g = 9.81; %ms2
    % % to = 0.05; %Nm
    Ix = 0.0030842; %kg.m2
    Iy = 0.0030842; %kg.m2
    Iz = 0.0032315; %kg.m2
    % Ir = 1E-4; %kg.m2
    U1 = T1+T2+T3+T4;
    U2 = l*(T2-T4);
    U3 = l*(T3-T1);
    U4 = T1-T2+T3-T4;

    x2dot=(U1*(sin(roll)*sin(yaw) + cos(roll)*cos(yaw)*sin(pitch)))/m;
    y2dot=-(U1*(cos(yaw)*sin(roll) - cos(roll)*sin(pitch)*sin(yaw)))/m;
    z2dot=(U1*cos(pitch)*cos(roll))/m - g;
    roll2dot=(Iy*pitch_dot*yaw_dot - Iz*pitch_dot*yaw_dot)/Ix + U2/Ix;
    pitch2dot=U3/Iy + (-Ix*roll_dot*yaw_dot + Iz*roll_dot*yaw_dot)/Iy;
    yaw2dot=U4/Iz + (Ix*pitch_dot*roll_dot - Iy*pitch_dot*roll_dot)/Iz;

% %% Gia lap ma sat theo cong thuc ma sat tuyen tinh voi he so cho truoc la
    FX_Friction     =  -  HS_MSKK * x_dot;
    FY_Friction     =  -  HS_MSKK * y_dot;
    FZ_Friction     =  -  HS_MSKK * z_dot;
    FR_Friction     =  -  HS_MSKK * roll_dot;
    FP_Friction     =  -  HS_MSKK * pitch_dot;
    FYaw_Friction   =  -  HS_MSKK * yaw_dot;
    FX_Limit        =     HS_MSKK /10;
    FY_Limit        =     HS_MSKK /10;
    FZ_Limit        =     HS_MSKK /10;
    FR_Limit        =     HS_MSKK /10;
    FP_Limit        =     HS_MSKK /10;
    FYaw_Limit      =     HS_MSKK /10;
    
    if(FX_Friction > FX_Limit)
        FX_Friction = FX_Limit;
    end
    if(FX_Friction < -FX_Limit)
        FX_Friction = -FX_Limit;
    end
    
    if(FY_Friction > FY_Limit)
        FY_Friction = FY_Limit;
    end
    if(FY_Friction < -FY_Limit)
        FY_Friction = -FY_Limit;
    end
    
    if(FZ_Friction > FZ_Limit)
        FZ_Friction = FZ_Limit;
    end
    if(FZ_Friction < -FZ_Limit)
        FZ_Friction = -FZ_Limit;
    end
    
    if(FR_Friction > FR_Limit)
        FR_Friction = FR_Limit;
    end
    if(FR_Friction < -FR_Limit)
        FR_Friction = -FR_Limit;
    end
    
    if(FP_Friction > FP_Limit)
        FP_Friction = FP_Limit;
    end
    if(FP_Friction < -FP_Limit)
        FP_Friction = -FP_Limit;
    end
    
    if(FYaw_Friction > FYaw_Limit)
        FYaw_Friction = FYaw_Limit;
    end
    if(FYaw_Friction < -FYaw_Limit)
        FYaw_Friction = -FYaw_Limit;
    end
    
    F_x2dot           = m*x2dot     - FX_Friction;
    if((m*x2dot)*(F_x2dot)<=0)
        F_x2dot     = m*x2dot;
    end
    F_y2dot           = m*y2dot     - FY_Friction;
    if((m*y2dot)*(F_y2dot)<=0)
        F_y2dot     = m*y2dot;
    end
    F_z2dot           = m*z2dot     - FZ_Friction;
    if((m*z2dot)*(F_z2dot)<=0)
        F_z2dot     = m*z2dot;
    end
    F_roll2dot        = m*roll2dot  - FR_Friction;
    if((m*roll2dot)*(F_roll2dot)<=0)
        F_roll2dot  = m*roll2dot;
    end
    F_pitch2dot       = m*pitch2dot - FP_Friction;
    if((m*pitch2dot)*(F_pitch2dot)<=0)
        F_pitch2dot = m*pitch2dot;
    end
    F_yaw2dot         = m*yaw2dot   - FYaw_Friction;
    if((m*yaw2dot)*(F_yaw2dot)<=0)
        F_yaw2dot   = m*yaw2dot;
    end

    x2dot           = F_x2dot/m;
    y2dot           = F_y2dot/m;
    z2dot           = F_z2dot/m;
    roll2dot        = F_roll2dot/m;
    pitch2dot       = F_pitch2dot/m;
    yaw2dot         = F_yaw2dot/m;
end
